simulink model "gap_generation_platoon"  (R2019a)
settings: Solver=VariableStepAuto  StartTime=0.0  StopTime=50  RelTol=1e-3
libraries: simulink x68, powerlib_meascontrol x7, autolibshared x7
(part 2 of 3)

== system gap_generation_platoon/p2 ==
  leaderStates : Inport
  virtualLeaderStates : Inport  Port=2
  lcFlag : Inport  Port=3
  activate ACC-v : Inport  Port=4
  ACC : Subsystem
  ACC-v : Subsystem
  AND : Logic  IconShape=distinctive  AllPortsSameDT=off  OutDataTypeStr=boolean
  Bus Creator : BusCreator  Inputs=4
  Bus Selector : BusSelector  OutputSignals=InertFrm.RearAxl.Disp.X,InertFrm.RearAxl.Disp.Y,InertFrm.RearAxl.Vel.Xdot
  Constant : Constant  Value=0
  Constant1 : Constant  Value=maxAcceleration+1
  Detect steady state : Subsystem
  Gain : Gain  Gain=m/2
  Min : MinMax  Inputs=2
  Mux1 : Mux  Inputs=6
  On Delay : powerlib_meascontrol/Logic/On Delay  DelayType=On delay  delay=1  ic=0  Ts=0
      settings: SourceProductName=Simscape Electrical
  Scope1 : Scope  NumInputPorts=3
  Signal Specification : SignalSpecification  Dimensions=1
  Switch : Switch  Criteria=u2 > Threshold
  Terminator : Terminator
  Triggered Subsystem : Subsystem  TreatAsAtomicUnit=on
  Vehicle Body 3DOF Single Track : autolibshared/Vehicle Body 3DOF Single Track  trackMode=Single (bicycle)  inputMode=External longitudinal forces  frontSteerMode=on  rearSteerMode=off  windMode=off  muMode=off  extFMode=off  extMMode=off  extXo=off  extpsio=off  extxdoto=off  extro=off  extYo=off  extTamb=off  extydoto=off  aMode=2  NF=2  NR=2  m=m  a=lf  b=lr  h=0.35  X_o=x0  xdot_o=vx0  CalphaMode=off  sigmaMode=on  d=0  w=[1.4,1.4]  Cy_f=12e3  Cy_r=11e3  sigma_f=.1  sigma_r=.1  alpha_f_brk=[-.1 .1]  Cy_f_data=[-9e3 9e3]  alpha_r_brk=[-.1 .1]  Cy_r_data=[-9e3 9e3]  Y_o=y0  ydot_o=0  Izz=4000  psi_o=0  r_o=0  Af=2  Cd=.3  Cl=.1  Cpm=.1  beta_w=[0:0.01:0.3]  Cs=[0:0.03:0.9]  Cym=[0:0.01:0.3]  Pabs=101325  Tair=273  g=9.81  mu=1  xdot_tol=.01  Fznom=5000  Fxtire_sat=7e4  Fytire_sat=7e4  longOff=0  latOff=0  vertOff=0  wrapAng=off
      settings: SourceProductName=Powertrain Blockset  SourceProductBaseCode=PW
  states : Outport
  errors : Outport  Port=2
  gap : Outport  Port=3
  virtualErrors : Outport  Port=4
  virtualGap : Outport  Port=5
  gapRequest : Outport  Port=6
  wires:
  Detect steady state/1(Out1) -> AND/1
  Triggered Subsystem/1(Out1) -> gapRequest/1
  On Delay/1 -> AND/2, Triggered Subsystem/1(In1)
  AND/1 -> Triggered Subsystem/Trigger
  Constant1/1 -> Switch/3
  activate ACC-v/1 -> Detect steady state/3(ACC-v active), ACC-v/3(activate), Switch/2
  Signal Specification/1 -> Gain/1, Bus Creator/4
  Bus Selector/2 -> Bus Creator/2  "<Y>"
  ACC-v/3(gap) -> virtualGap/1
  ACC-v/2(errors) -> virtualErrors/1, Detect steady state/2(virtual errors)
  ACC-v/1(u) -> Switch/1
  Switch/1 -> Min/2, Scope1/2  "acc-v"
  lcFlag/1 -> ACC/3(lcFlag), On Delay/1, ACC-v/4(lcFlag)
  ACC/2(errors) -> Detect steady state/1(errors), errors/1
  virtualLeaderStates/1 -> ACC-v/2(leaderStates)
  leaderStates/1 -> ACC/2(leaderStates)
  Bus Creator/1 -> states/1, ACC-v/1(currentStates), ACC/1(currentStates)
  ACC/3(gap) -> gap/1
  Mux1/1 -> Terminator/1
  Vehicle Body 3DOF Single Track/7 -> Mux1/6
  Vehicle Body 3DOF Single Track/6 -> Mux1/5
  Vehicle Body 3DOF Single Track/5 -> Mux1/4
  Vehicle Body 3DOF Single Track/2 -> Mux1/1
  Vehicle Body 3DOF Single Track/3 -> Mux1/2
  Vehicle Body 3DOF Single Track/4 -> Mux1/3
  Vehicle Body 3DOF Single Track/1 -> Bus Selector/1
  Constant/1 -> Vehicle Body 3DOF Single Track/1
  Gain/1 -> Vehicle Body 3DOF Single Track/2, Vehicle Body 3DOF Single Track/3
  ACC/1(u) -> Min/1, Scope1/1  "acc"
  Min/1 -> Signal Specification/1, Scope1/3  "u"
  Bus Selector/1 -> Bus Creator/1  "<X>"
  Bus Selector/3 -> Bus Creator/3  "<Xdot>"

== system gap_generation_platoon/p3 ==
  leaderStates : Inport
  virtualLeaderStates : Inport  Port=2
  lcFlag : Inport  Port=3
  activate ACC-v : Inport  Port=4
  ACC : Subsystem
  ACC-v : Subsystem
  AND : Logic  IconShape=distinctive  AllPortsSameDT=off  OutDataTypeStr=boolean
  Bus Creator : BusCreator  Inputs=4
  Bus Selector : BusSelector  OutputSignals=InertFrm.RearAxl.Disp.X,InertFrm.RearAxl.Disp.Y,InertFrm.RearAxl.Vel.Xdot
  Constant : Constant  Value=0
  Constant1 : Constant  Value=maxAcceleration+1
  Detect steady state : Subsystem
  Gain : Gain  Gain=m/2
  Min : MinMax  Inputs=2
  Mux1 : Mux  Inputs=6
  On Delay : powerlib_meascontrol/Logic/On Delay  DelayType=On delay  delay=1  ic=0  Ts=0
      settings: SourceProductName=Simscape Electrical
  Scope1 : Scope  NumInputPorts=3
  Signal Specification : SignalSpecification  Dimensions=1
  Switch : Switch  Criteria=u2 > Threshold
  Terminator : Terminator
  Triggered Subsystem : Subsystem  TreatAsAtomicUnit=on
  Vehicle Body 3DOF Single Track : autolibshared/Vehicle Body 3DOF Single Track  trackMode=Single (bicycle)  inputMode=External longitudinal forces  frontSteerMode=on  rearSteerMode=off  windMode=off  muMode=off  extFMode=off  extMMode=off  extXo=off  extpsio=off  extxdoto=off  extro=off  extYo=off  extTamb=off  extydoto=off  aMode=2  NF=2  NR=2  m=m  a=lf  b=lr  h=0.35  X_o=x0  xdot_o=vx0  CalphaMode=off  sigmaMode=on  d=0  w=[1.4,1.4]  Cy_f=12e3  Cy_r=11e3  sigma_f=.1  sigma_r=.1  alpha_f_brk=[-.1 .1]  Cy_f_data=[-9e3 9e3]  alpha_r_brk=[-.1 .1]  Cy_r_data=[-9e3 9e3]  Y_o=y0  ydot_o=0  Izz=4000  psi_o=0  r_o=0  Af=2  Cd=.3  Cl=.1  Cpm=.1  beta_w=[0:0.01:0.3]  Cs=[0:0.03:0.9]  Cym=[0:0.01:0.3]  Pabs=101325  Tair=273  g=9.81  mu=1  xdot_tol=.01  Fznom=5000  Fxtire_sat=7e4  Fytire_sat=7e4  longOff=0  latOff=0  vertOff=0  wrapAng=off
      settings: SourceProductName=Powertrain Blockset  SourceProductBaseCode=PW
  states : Outport
  errors : Outport  Port=2
  gap : Outport  Port=3
  virtualErrors : Outport  Port=4
  virtualGap : Outport  Port=5
  gapRequest : Outport  Port=6
  wires:
  Bus Selector/3 -> Bus Creator/3  "<Xdot>"
  Bus Selector/1 -> Bus Creator/1  "<X>"
  Min/1 -> Scope1/3, Signal Specification/1  "u"
  ACC/1(u) -> Scope1/1, Min/1  "acc"
  Gain/1 -> Vehicle Body 3DOF Single Track/3, Vehicle Body 3DOF Single Track/2
  Constant/1 -> Vehicle Body 3DOF Single Track/1
  Vehicle Body 3DOF Single Track/1 -> Bus Selector/1
  Vehicle Body 3DOF Single Track/4 -> Mux1/3
  Vehicle Body 3DOF Single Track/3 -> Mux1/2
  Vehicle Body 3DOF Single Track/2 -> Mux1/1
  Vehicle Body 3DOF Single Track/5 -> Mux1/4
  Vehicle Body 3DOF Single Track/6 -> Mux1/5
  Vehicle Body 3DOF Single Track/7 -> Mux1/6
  Mux1/1 -> Terminator/1
  ACC/3(gap) -> gap/1
  Bus Creator/1 -> ACC/1(currentStates), ACC-v/1(currentStates), states/1
  leaderStates/1 -> ACC/2(leaderStates)
  virtualLeaderStates/1 -> ACC-v/2(leaderStates)
  ACC/2(errors) -> errors/1, Detect steady state/1(errors)
  lcFlag/1 -> ACC-v/4(lcFlag), On Delay/1, ACC/3(lcFlag)
  Switch/1 -> Scope1/2, Min/2  "acc-v"
  ACC-v/1(u) -> Switch/1
  ACC-v/2(errors) -> Detect steady state/2(virtual errors), virtualErrors/1
  ACC-v/3(gap) -> virtualGap/1
  Bus Selector/2 -> Bus Creator/2  "<Y>"
  Signal Specification/1 -> Bus Creator/4, Gain/1
  activate ACC-v/1 -> Switch/2, ACC-v/3(activate), Detect steady state/3(ACC-v active)
  Constant1/1 -> Switch/3
  AND/1 -> Triggered Subsystem/Trigger
  On Delay/1 -> Triggered Subsystem/1(In1), AND/2
  Triggered Subsystem/1(Out1) -> gapRequest/1
  Detect steady state/1(Out1) -> AND/1

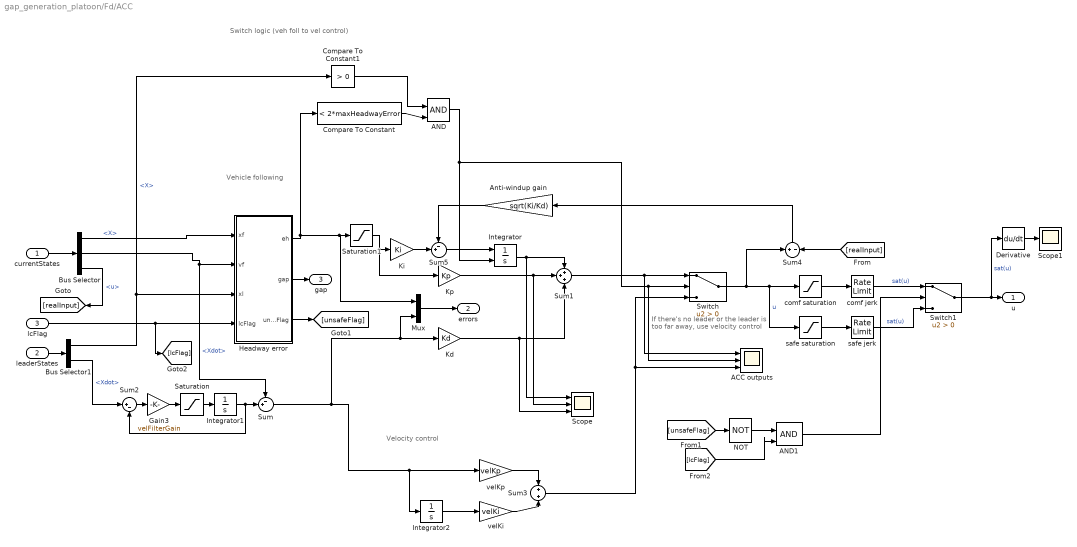
== system gap_generation_platoon/Fd/ACC ==
  note: Vehicle following
  note: Switch logic (veh foll to vel control)
  note: Velocity control
  note: If there's no leader or the leader
      | is too far away, use velocity control
  currentStates : Inport
  leaderStates : Inport  Port=2
  lcFlag : Inport  Port=3
  ACC outputs : Scope  NumInputPorts=3
  AND : Logic  IconShape=distinctive  AllPortsSameDT=off  OutDataTypeStr=boolean
  AND1 : Logic  IconShape=distinctive  AllPortsSameDT=off  OutDataTypeStr=boolean
  Anti-windup gain : Gain  Gain=sqrt(Ki/Kd)
  Bus Selector : BusSelector  OutputSignals=X,Xdot,u
  Bus Selector1 : BusSelector  OutputSignals=X,Xdot
  Compare To Constant : simulink/Logic and Bit Operations/Compare To Constant  relop=<  const=2*maxHeadwayError  OutDataTypeStr=boolean
  Compare To Constant1 : simulink/Logic and Bit Operations/Compare To Constant  relop=>  const=0  OutDataTypeStr=boolean
  Derivative : Derivative
  Gain3 : Gain  Gain=velFilterGain
  Headway error : Subsystem
  Integrator : Integrator  ExternalReset=either
  Integrator1 : Integrator  InitialCondition=vx0
  Integrator2 : Integrator
  Kd : Gain  Gain=Kd
  Ki : Gain  Gain=Ki
  Kp : Gain  Gain=Kp
  Mux : Mux  Inputs=2
  NOT : Logic  Operator=NOT  IconShape=distinctive  AllPortsSameDT=off  OutDataTypeStr=boolean
  Saturation : Saturate  UpperLimit=maxAcceleration  LowerLimit=minAcceleration
  Saturation1 : Saturate  UpperLimit=maxHeadwayError  LowerLimit=minHeadwayError
  Scope : Scope  NumInputPorts=3
  Scope1 : Scope
  Sum : Sum  Inputs=-+|
  Sum1 : Sum  Inputs=+++
  Sum2 : Sum  Inputs=|+-
  Sum3 : Sum
  Sum4 : Sum  Inputs=+-
  Sum5 : Sum  Inputs=-+|
  Switch : Switch  Criteria=u2 > Threshold
  Switch1 : Switch  Criteria=u2 > Threshold
  comf jerk : RateLimiter  RisingSlewLimit=10  FallingSlewLimit=-10  SampleTimeMode=inherited
  comf saturation : Saturate  UpperLimit=maxAcceleration/2  LowerLimit=minAcceleration/4
  safe jerk : RateLimiter  RisingSlewLimit=maxJerk  FallingSlewLimit=minJerk  SampleTimeMode=inherited
  safe saturation : Saturate  UpperLimit=maxAcceleration  LowerLimit=minAcceleration
  velKi : Gain  Gain=velKi
  velKp : Gain  Gain=velKp
  u : Outport
  errors : Outport  Port=2
  gap : Outport  Port=3
  wires:
  Headway error/1(eh) -> Saturation1/1, Mux/1, Compare To Constant/1
  Bus Selector/2 -> Headway error/2(vf), Sum/1  "<Xdot>"
  Kd/1 -> Scope/3, Sum1/3
  Kp/1 -> Scope/2, Sum1/2
  Gain3/1 -> Saturation/1
  Saturation/1 -> Integrator1/1
  Integrator1/1 -> Sum2/2, Sum/2
  Bus Selector1/2 -> Sum2/1  "<Xdot>"
  Sum2/1 -> Gain3/1
  Saturation1/1 -> Kp/1, Ki/1
  Headway error/2("gap ") -> gap/1
  Integrator2/1 -> velKi/1
  velKi/1 -> Sum3/2
  Switch/1 -> Sum4/1, safe saturation/1, comf saturation/1  "u"
  Sum1/1 -> Switch/1, ACC outputs/1
  Sum3/1 -> ACC outputs/3, Switch/3
  Sum/1 -> Mux/2, Kd/1, velKp/1, Integrator2/1
  Mux/1 -> errors/1
  Sum4/1 -> Anti-windup gain/1
  Sum5/1 -> Integrator/1
  Switch1/1 -> Derivative/1, u/1  "sat(u)"
  velKp/1 -> Sum3/1
  Ki/1 -> Sum5/2
  Integrator/1 -> Sum1/1, Scope/1
  Anti-windup gain/1 -> Sum5/1
  AND/1 -> Integrator/2, Switch/2, ACC outputs/2
  Compare To Constant/1 -> AND/2
  Compare To Constant1/1 -> AND/1
  lcFlag/1 -> [lcFlag], Headway error/4(lcFlag)
  currentStates/1 -> Bus Selector/1
  Bus Selector/1 -> Headway error/1(xf)  "<X>"
  leaderStates/1 -> Bus Selector1/1
  Bus Selector1/1 -> Compare To Constant1/1, Headway error/3(xl)  "<X>"
  Bus Selector/3 -> [realInput]  "<u>"
  [realInput] -> Sum4/2
  Headway error/3(unsafeFlag) -> [unsafeFlag]
  [unsafeFlag] -> NOT/1
  NOT/1 -> AND1/1
  [lcFlag] -> AND1/2
  AND1/1 -> Switch1/2
  safe saturation/1 -> safe jerk/1
  comf saturation/1 -> comf jerk/1
  safe jerk/1 -> Switch1/3  "sat(u)"
  comf jerk/1 -> Switch1/1  "sat(u)"
  Derivative/1 -> Scope1/1

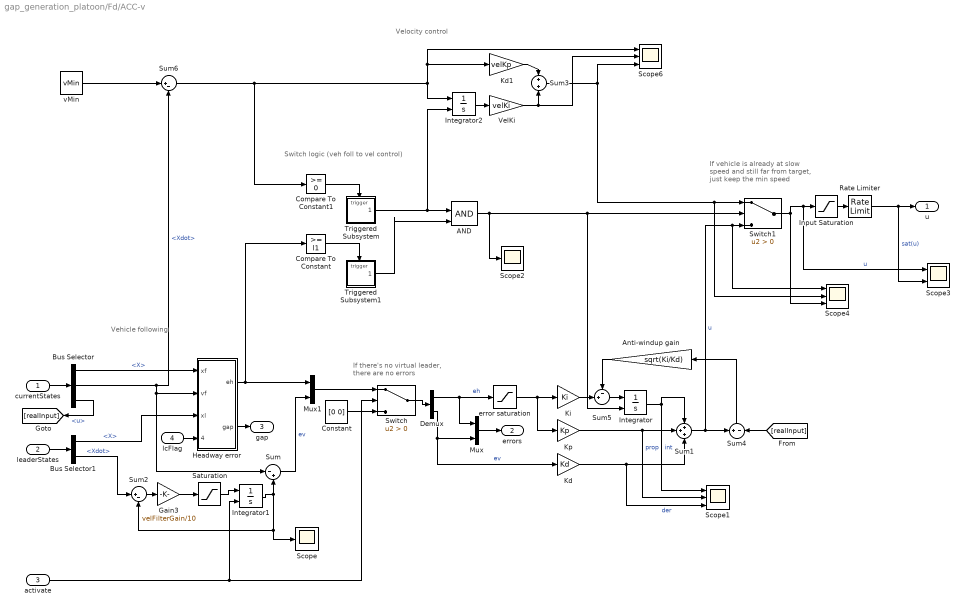
== system gap_generation_platoon/Fd/ACC-v ==
  note: Vehicle following
  note: Switch logic (veh foll to vel control)
  note: Velocity control
  note: If vehicle is already at slow
      | speed and still far from target,
      | just keep the min speed
  note: If there's no virtual leader,
      | there are no errors
  currentStates : Inport
  leaderStates : Inport  Port=2
  activate : Inport  Port=3
  lcFlag : Inport  Port=4
  AND : Logic  IconShape=distinctive  AllPortsSameDT=off  OutDataTypeStr=boolean
  Anti-windup gain : Gain  Gain=sqrt(Ki/Kd)
  Bus Selector : BusSelector  OutputSignals=X,Xdot,u
  Bus Selector1 : BusSelector  OutputSignals=X,Xdot
  Compare To Constant : simulink/Logic and Bit Operations/Compare To Constant  relop=>=  const=l1  OutDataTypeStr=boolean
  Compare To Constant1 : simulink/Logic and Bit Operations/Compare To Constant  relop=>=  const=0  OutDataTypeStr=boolean
  Constant : Constant  Value=[0 0]
  Demux : Demux  Outputs=2
  Gain3 : Gain  Gain=velFilterGain/10
  Headway error : Subsystem
  Input Saturation : Saturate  UpperLimit=maxAcceleration/2  LowerLimit=minAcceleration/4
  Integrator : Integrator  ExternalReset=falling
  Integrator1 : Integrator  ExternalReset=rising  InitialCondition=vx0
  Integrator2 : Integrator  ExternalReset=rising
  Kd : Gain  Gain=Kd
  Kd1 : Gain  Gain=velKp
  Ki : Gain  Gain=Ki
  Kp : Gain  Gain=Kp
  Mux : Mux  Inputs=2
  Mux1 : Mux  Inputs=2
  Rate Limiter : RateLimiter  RisingSlewLimit=10  FallingSlewLimit=-10  SampleTimeMode=inherited
  Saturation : Saturate  UpperLimit=maxAcceleration  LowerLimit=minAcceleration
  Scope : Scope
  Scope1 : Scope  NumInputPorts=3
  Scope2 : Scope
  Scope3 : Scope  NumInputPorts=2
  Scope4 : Scope  NumInputPorts=3
  Scope6 : Scope  NumInputPorts=3
  Sum : Sum  Inputs=|-+
  Sum1 : Sum  Inputs=+++
  Sum2 : Sum  Inputs=|+-
  Sum3 : Sum
  Sum4 : Sum  Inputs=+-
  Sum5 : Sum  Inputs=-+|
  Sum6 : Sum  Inputs=|+-
  Switch : Switch  Criteria=u2 > Threshold
  Switch1 : Switch  Criteria=u2 > Threshold
  Triggered Subsystem : Subsystem  TreatAsAtomicUnit=on
  Triggered Subsystem1 : Subsystem  TreatAsAtomicUnit=on
  VelKi : Gain  Gain=velKi
  error saturation : Saturate  UpperLimit=maxHeadwayError  LowerLimit=minHeadwayError/10
  vMin : Constant  Value=vMin
  u : Outport
  errors : Outport  Port=2
  gap : Outport  Port=3
  wires:
  Headway error/1(eh) -> Mux1/1, Compare To Constant/1
  Kd/1 -> Scope1/3, Sum1/3  "der"
  Kp/1 -> Scope1/2, Sum1/2  "prop"
  Gain3/1 -> Saturation/1
  Saturation/1 -> Integrator1/1
  Integrator1/1 -> Scope/1, Sum2/2, Sum/2
  Bus Selector1/2 -> Sum2/1  "<Xdot>"
  Sum2/1 -> Gain3/1
  Demux/1 -> error saturation/1, Mux/1  "eh"
  Headway error/2("gap ") -> gap/1
  Sum1/1 -> Scope4/1, Switch1/3, Sum4/1  "u"
  Sum/1 -> Mux1/2  "ev"
  Mux/1 -> errors/1
  Input Saturation/1 -> Rate Limiter/1
  Integrator/1 -> Sum1/1, Scope1/1  "int"
  Sum4/1 -> Anti-windup gain/1
  Ki/1 -> Sum5/2
  Anti-windup gain/1 -> Sum5/1
  Demux/2 -> Mux/2, Kd/1  "ev"
  Switch/1 -> Demux/1
  Mux1/1 -> Switch/1
  activate/1 -> Switch/2, Integrator1/2
  Constant/1 -> Switch/3
  Rate Limiter/1 -> Scope3/2, u/1  "sat(u)"
  Compare To Constant1/1 -> Triggered Subsystem/Trigger
  Compare To Constant/1 -> Triggered Subsystem1/Trigger
  Sum6/1 -> Scope6/1, Kd1/1, Integrator2/1, Compare To Constant1/1
  Sum3/1 -> Scope6/3, Scope4/2, Switch1/1
  Integrator2/1 -> VelKi/1
  Kd1/1 -> Sum3/1
  VelKi/1 -> Scope6/2, Sum3/2
  vMin/1 -> Sum6/1
  Switch1/1 -> Scope3/1, Input Saturation/1, Scope4/3  "u"
  error saturation/1 -> Kp/1, Ki/1
  Sum5/1 -> Integrator/1
  Triggered Subsystem/1(Out1) -> AND/1, Integrator2/2
  [realInput] -> Sum4/2
  currentStates/1 -> Bus Selector/1
  Bus Selector/1 -> Headway error/1(xf)  "<X>"
  Bus Selector/2 -> Sum6/2, Headway error/2(vf), Sum/1  "<Xdot>"
  leaderStates/1 -> Bus Selector1/1
  Bus Selector1/1 -> Headway error/3(xl)  "<X>"
  Bus Selector/3 -> [realInput]  "<u>"
  lcFlag/1 -> Headway error/4(lcFlag)
  Triggered Subsystem1/1(Out1) -> AND/2
  AND/1 -> Switch1/2, Integrator/2, Scope2/1

== system gap_generation_platoon/Fd/Triggered Subsystem ==
  In1 : Inport
  Trigger : TriggerPort  VariantControl=Variant
  Out1 : Outport
  wires:
  In1/1 -> Out1/1

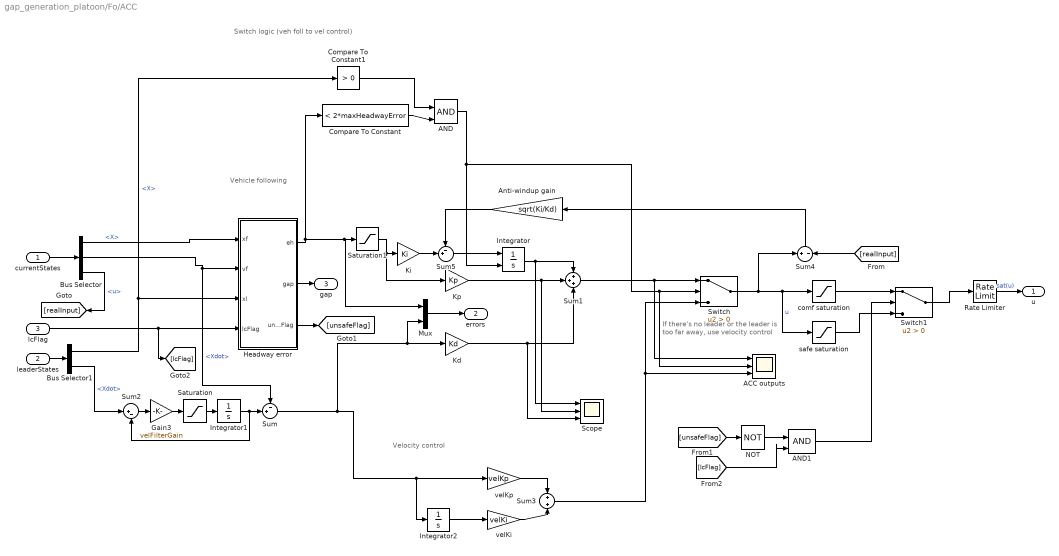
== system gap_generation_platoon/Fo/ACC ==
  note: If there's no leader or the leader
      | is too far away, use velocity control
  note: Velocity control
  note: Switch logic (veh foll to vel control)
  note: Vehicle following
  currentStates : Inport
  leaderStates : Inport  Port=2
  lcFlag : Inport  Port=3
  ACC outputs : Scope  NumInputPorts=3
  AND : Logic  IconShape=distinctive  AllPortsSameDT=off  OutDataTypeStr=boolean
  AND1 : Logic  IconShape=distinctive  AllPortsSameDT=off  OutDataTypeStr=boolean
  Anti-windup gain : Gain  Gain=sqrt(Ki/Kd)
  Bus Selector : BusSelector  OutputSignals=X,Xdot,u
  Bus Selector1 : BusSelector  OutputSignals=X,Xdot
  Compare To Constant : simulink/Logic and Bit Operations/Compare To Constant  relop=<  const=2*maxHeadwayError  OutDataTypeStr=boolean
  Compare To Constant1 : simulink/Logic and Bit Operations/Compare To Constant  relop=>  const=0  OutDataTypeStr=boolean
  Gain3 : Gain  Gain=velFilterGain
  Headway error : Subsystem
  Integrator : Integrator  ExternalReset=either
  Integrator1 : Integrator  InitialCondition=vx0
  Integrator2 : Integrator
  Kd : Gain  Gain=Kd
  Ki : Gain  Gain=Ki
  Kp : Gain  Gain=Kp
  Mux : Mux  Inputs=2
  NOT : Logic  Operator=NOT  IconShape=distinctive  AllPortsSameDT=off  OutDataTypeStr=boolean
  Rate Limiter : RateLimiter  RisingSlewLimit=maxJerk  FallingSlewLimit=minJerk  SampleTimeMode=inherited
  Saturation : Saturate  UpperLimit=maxAcceleration  LowerLimit=minAcceleration
  Saturation1 : Saturate  UpperLimit=maxHeadwayError  LowerLimit=minHeadwayError
  Scope : Scope  NumInputPorts=3
  Sum : Sum  Inputs=-+|
  Sum1 : Sum  Inputs=+++
  Sum2 : Sum  Inputs=|+-
  Sum3 : Sum
  Sum4 : Sum  Inputs=+-
  Sum5 : Sum  Inputs=-+|
  Switch : Switch  Criteria=u2 > Threshold
  Switch1 : Switch  Criteria=u2 > Threshold
  comf saturation : Saturate  UpperLimit=maxAcceleration/2  LowerLimit=minAcceleration/4
  safe saturation : Saturate  UpperLimit=maxAcceleration  LowerLimit=minAcceleration
  velKi : Gain  Gain=velKi
  velKp : Gain  Gain=velKp
  u : Outport
  errors : Outport  Port=2
  gap : Outport  Port=3
  wires:
  comf saturation/1 -> Switch1/1
  safe saturation/1 -> Switch1/3
  Switch1/1 -> Rate Limiter/1
  AND1/1 -> Switch1/2
  [lcFlag] -> AND1/2
  NOT/1 -> AND1/1
  [unsafeFlag] -> NOT/1
  Headway error/3(unsafeFlag) -> [unsafeFlag]
  [realInput] -> Sum4/2
  Bus Selector/3 -> [realInput]  "<u>"
  Bus Selector1/1 -> Headway error/3(xl), Compare To Constant1/1  "<X>"
  leaderStates/1 -> Bus Selector1/1
  Bus Selector/1 -> Headway error/1(xf)  "<X>"
  currentStates/1 -> Bus Selector/1
  lcFlag/1 -> Headway error/4(lcFlag), [lcFlag]
  Compare To Constant1/1 -> AND/1
  Compare To Constant/1 -> AND/2
  AND/1 -> ACC outputs/2, Switch/2, Integrator/2
  Anti-windup gain/1 -> Sum5/1
  Integrator/1 -> Scope/1, Sum1/1
  Ki/1 -> Sum5/2
  velKp/1 -> Sum3/1
  Rate Limiter/1 -> u/1  "sat(u)"
  Sum5/1 -> Integrator/1
  Sum4/1 -> Anti-windup gain/1
  Mux/1 -> errors/1
  Sum/1 -> Integrator2/1, velKp/1, Kd/1, Mux/2
  Sum3/1 -> Switch/3, ACC outputs/3
  Sum1/1 -> ACC outputs/1, Switch/1
  Switch/1 -> comf saturation/1, safe saturation/1, Sum4/1  "u"
  velKi/1 -> Sum3/2
  Integrator2/1 -> velKi/1
  Headway error/2("gap ") -> gap/1
  Saturation1/1 -> Ki/1, Kp/1
  Sum2/1 -> Gain3/1
  Bus Selector1/2 -> Sum2/1  "<Xdot>"
  Integrator1/1 -> Sum/2, Sum2/2
  Saturation/1 -> Integrator1/1
  Gain3/1 -> Saturation/1
  Kp/1 -> Sum1/2, Scope/2
  Kd/1 -> Sum1/3, Scope/3
  Bus Selector/2 -> Sum/1, Headway error/2(vf)  "<Xdot>"
  Headway error/1(eh) -> Compare To Constant/1, Mux/1, Saturation1/1

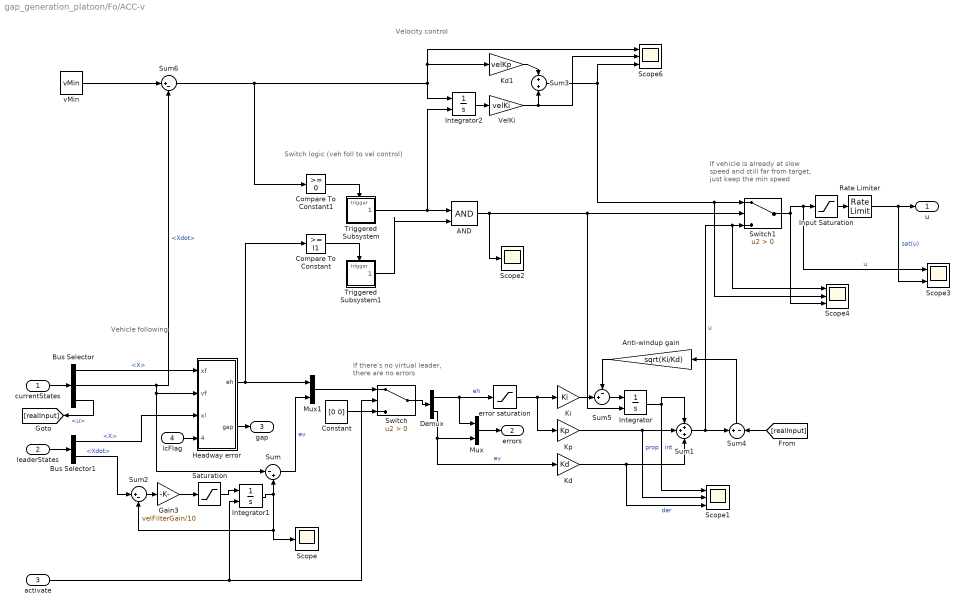
== system gap_generation_platoon/Fo/ACC-v ==
  note: If there's no virtual leader,
      | there are no errors
  note: If vehicle is already at slow
      | speed and still far from target,
      | just keep the min speed
  note: Velocity control
  note: Switch logic (veh foll to vel control)
  note: Vehicle following
  currentStates : Inport
  leaderStates : Inport  Port=2
  activate : Inport  Port=3
  lcFlag : Inport  Port=4
  AND : Logic  IconShape=distinctive  AllPortsSameDT=off  OutDataTypeStr=boolean
  Anti-windup gain : Gain  Gain=sqrt(Ki/Kd)
  Bus Selector : BusSelector  OutputSignals=X,Xdot,u
  Bus Selector1 : BusSelector  OutputSignals=X,Xdot
  Compare To Constant : simulink/Logic and Bit Operations/Compare To Constant  relop=>=  const=l1  OutDataTypeStr=boolean
  Compare To Constant1 : simulink/Logic and Bit Operations/Compare To Constant  relop=>=  const=0  OutDataTypeStr=boolean
  Constant : Constant  Value=[0 0]
  Demux : Demux  Outputs=2
  Gain3 : Gain  Gain=velFilterGain/10
  Headway error : Subsystem
  Input Saturation : Saturate  UpperLimit=maxAcceleration/2  LowerLimit=minAcceleration/4
  Integrator : Integrator  ExternalReset=falling
  Integrator1 : Integrator  ExternalReset=rising  InitialCondition=vx0
  Integrator2 : Integrator  ExternalReset=rising
  Kd : Gain  Gain=Kd
  Kd1 : Gain  Gain=velKp
  Ki : Gain  Gain=Ki
  Kp : Gain  Gain=Kp
  Mux : Mux  Inputs=2
  Mux1 : Mux  Inputs=2
  Rate Limiter : RateLimiter  RisingSlewLimit=maxJerk/2  FallingSlewLimit=minJerk/3  SampleTimeMode=inherited
  Saturation : Saturate  UpperLimit=maxAcceleration  LowerLimit=minAcceleration
  Scope : Scope
  Scope1 : Scope  NumInputPorts=3
  Scope2 : Scope
  Scope3 : Scope  NumInputPorts=2
  Scope4 : Scope  NumInputPorts=3
  Scope6 : Scope  NumInputPorts=3
  Sum : Sum  Inputs=|-+
  Sum1 : Sum  Inputs=+++
  Sum2 : Sum  Inputs=|+-
  Sum3 : Sum
  Sum4 : Sum  Inputs=+-
  Sum5 : Sum  Inputs=-+|
  Sum6 : Sum  Inputs=|+-
  Switch : Switch  Criteria=u2 > Threshold
  Switch1 : Switch  Criteria=u2 > Threshold
  Triggered Subsystem : Subsystem  TreatAsAtomicUnit=on
  Triggered Subsystem1 : Subsystem  TreatAsAtomicUnit=on
  VelKi : Gain  Gain=velKi
  error saturation : Saturate  UpperLimit=maxHeadwayError  LowerLimit=minHeadwayError/10
  vMin : Constant  Value=vMin
  u : Outport
  errors : Outport  Port=2
  gap : Outport  Port=3
  wires:
  AND/1 -> Scope2/1, Integrator/2, Switch1/2
  Triggered Subsystem1/1(Out1) -> AND/2
  lcFlag/1 -> Headway error/4(lcFlag)
  Bus Selector/3 -> [realInput]  "<u>"
  Bus Selector1/1 -> Headway error/3(xl)  "<X>"
  leaderStates/1 -> Bus Selector1/1
  Bus Selector/2 -> Sum/1, Headway error/2(vf), Sum6/2  "<Xdot>"
  Bus Selector/1 -> Headway error/1(xf)  "<X>"
  currentStates/1 -> Bus Selector/1
  [realInput] -> Sum4/2
  Triggered Subsystem/1(Out1) -> Integrator2/2, AND/1
  Sum5/1 -> Integrator/1
  error saturation/1 -> Ki/1, Kp/1
  Switch1/1 -> Scope4/3, Input Saturation/1, Scope3/1  "u"
  vMin/1 -> Sum6/1
  VelKi/1 -> Sum3/2, Scope6/2
  Kd1/1 -> Sum3/1
  Integrator2/1 -> VelKi/1
  Sum3/1 -> Switch1/1, Scope4/2, Scope6/3
  Sum6/1 -> Compare To Constant1/1, Integrator2/1, Kd1/1, Scope6/1
  Compare To Constant/1 -> Triggered Subsystem1/Trigger
  Compare To Constant1/1 -> Triggered Subsystem/Trigger
  Rate Limiter/1 -> u/1, Scope3/2  "sat(u)"
  Constant/1 -> Switch/3
  activate/1 -> Integrator1/2, Switch/2
  Mux1/1 -> Switch/1
  Switch/1 -> Demux/1
  Demux/2 -> Kd/1, Mux/2  "ev"
  Anti-windup gain/1 -> Sum5/1
  Ki/1 -> Sum5/2
  Sum4/1 -> Anti-windup gain/1
  Integrator/1 -> Scope1/1, Sum1/1  "int"
  Input Saturation/1 -> Rate Limiter/1
  Mux/1 -> errors/1
  Sum/1 -> Mux1/2  "ev"
  Sum1/1 -> Sum4/1, Switch1/3, Scope4/1  "u"
  Headway error/2("gap ") -> gap/1
  Demux/1 -> Mux/1, error saturation/1  "eh"
  Sum2/1 -> Gain3/1
  Bus Selector1/2 -> Sum2/1  "<Xdot>"
  Integrator1/1 -> Sum/2, Sum2/2, Scope/1
  Saturation/1 -> Integrator1/1
  Gain3/1 -> Saturation/1
  Kp/1 -> Sum1/2, Scope1/2  "prop"
  Kd/1 -> Sum1/3, Scope1/3  "der"
  Headway error/1(eh) -> Compare To Constant/1, Mux1/1

== system gap_generation_platoon/Fo/Triggered Subsystem ==
  In1 : Inport
  Trigger : TriggerPort  VariantControl=Variant
  Out1 : Outport
  wires:
  In1/1 -> Out1/1

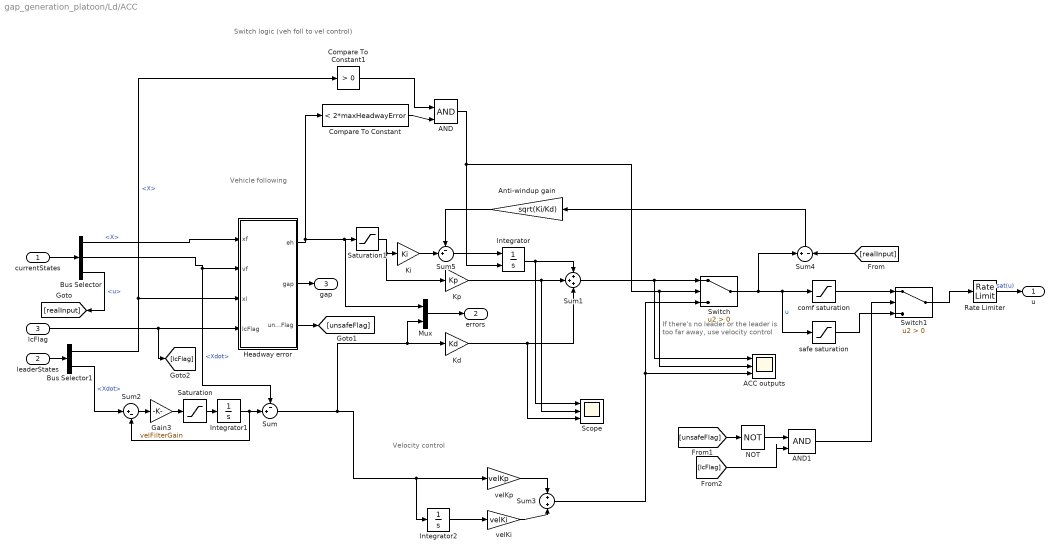
== system gap_generation_platoon/Ld/ACC ==
  note: If there's no leader or the leader
      | is too far away, use velocity control
  note: Velocity control
  note: Switch logic (veh foll to vel control)
  note: Vehicle following
  currentStates : Inport
  leaderStates : Inport  Port=2
  lcFlag : Inport  Port=3
  ACC outputs : Scope  NumInputPorts=3
  AND : Logic  IconShape=distinctive  AllPortsSameDT=off  OutDataTypeStr=boolean
  AND1 : Logic  IconShape=distinctive  AllPortsSameDT=off  OutDataTypeStr=boolean
  Anti-windup gain : Gain  Gain=sqrt(Ki/Kd)
  Bus Selector : BusSelector  OutputSignals=X,Xdot,u
  Bus Selector1 : BusSelector  OutputSignals=X,Xdot
  Compare To Constant : simulink/Logic and Bit Operations/Compare To Constant  relop=<  const=2*maxHeadwayError  OutDataTypeStr=boolean
  Compare To Constant1 : simulink/Logic and Bit Operations/Compare To Constant  relop=>  const=0  OutDataTypeStr=boolean
  Gain3 : Gain  Gain=velFilterGain
  Headway error : Subsystem
  Integrator : Integrator  ExternalReset=either
  Integrator1 : Integrator  InitialCondition=vx0
  Integrator2 : Integrator
  Kd : Gain  Gain=Kd
  Ki : Gain  Gain=Ki
  Kp : Gain  Gain=Kp
  Mux : Mux  Inputs=2
  NOT : Logic  Operator=NOT  IconShape=distinctive  AllPortsSameDT=off  OutDataTypeStr=boolean
  Rate Limiter : RateLimiter  RisingSlewLimit=maxJerk  FallingSlewLimit=minJerk  SampleTimeMode=inherited
  Saturation : Saturate  UpperLimit=maxAcceleration  LowerLimit=minAcceleration
  Saturation1 : Saturate  UpperLimit=maxHeadwayError  LowerLimit=minHeadwayError
  Scope : Scope  NumInputPorts=3
  Sum : Sum  Inputs=-+|
  Sum1 : Sum  Inputs=+++
  Sum2 : Sum  Inputs=|+-
  Sum3 : Sum
  Sum4 : Sum  Inputs=+-
  Sum5 : Sum  Inputs=-+|
  Switch : Switch  Criteria=u2 > Threshold
  Switch1 : Switch  Criteria=u2 > Threshold
  comf saturation : Saturate  UpperLimit=maxAcceleration/2  LowerLimit=minAcceleration/4
  safe saturation : Saturate  UpperLimit=maxAcceleration  LowerLimit=minAcceleration
  velKi : Gain  Gain=velKi
  velKp : Gain  Gain=velKp
  u : Outport
  errors : Outport  Port=2
  gap : Outport  Port=3
  wires:
  comf saturation/1 -> Switch1/1
  safe saturation/1 -> Switch1/3
  Switch1/1 -> Rate Limiter/1
  AND1/1 -> Switch1/2
  [lcFlag] -> AND1/2
  NOT/1 -> AND1/1
  [unsafeFlag] -> NOT/1
  Headway error/3(unsafeFlag) -> [unsafeFlag]
  [realInput] -> Sum4/2
  Bus Selector/3 -> [realInput]  "<u>"
  Bus Selector1/1 -> Headway error/3(xl), Compare To Constant1/1  "<X>"
  leaderStates/1 -> Bus Selector1/1
  Bus Selector/1 -> Headway error/1(xf)  "<X>"
  currentStates/1 -> Bus Selector/1
  lcFlag/1 -> Headway error/4(lcFlag), [lcFlag]
  Compare To Constant1/1 -> AND/1
  Compare To Constant/1 -> AND/2
  AND/1 -> ACC outputs/2, Switch/2, Integrator/2
  Anti-windup gain/1 -> Sum5/1
  Integrator/1 -> Scope/1, Sum1/1
  Ki/1 -> Sum5/2
  velKp/1 -> Sum3/1
  Rate Limiter/1 -> u/1  "sat(u)"
  Sum5/1 -> Integrator/1
  Sum4/1 -> Anti-windup gain/1
  Mux/1 -> errors/1
  Sum/1 -> Integrator2/1, velKp/1, Kd/1, Mux/2
  Sum3/1 -> Switch/3, ACC outputs/3
  Sum1/1 -> ACC outputs/1, Switch/1
  Switch/1 -> comf saturation/1, safe saturation/1, Sum4/1  "u"
  velKi/1 -> Sum3/2
  Integrator2/1 -> velKi/1
  Headway error/2("gap ") -> gap/1
  Saturation1/1 -> Ki/1, Kp/1
  Sum2/1 -> Gain3/1
  Bus Selector1/2 -> Sum2/1  "<Xdot>"
  Integrator1/1 -> Sum/2, Sum2/2
  Saturation/1 -> Integrator1/1
  Gain3/1 -> Saturation/1
  Kp/1 -> Sum1/2, Scope/2
  Kd/1 -> Sum1/3, Scope/3
  Bus Selector/2 -> Sum/1, Headway error/2(vf)  "<Xdot>"
  Headway error/1(eh) -> Compare To Constant/1, Mux/1, Saturation1/1

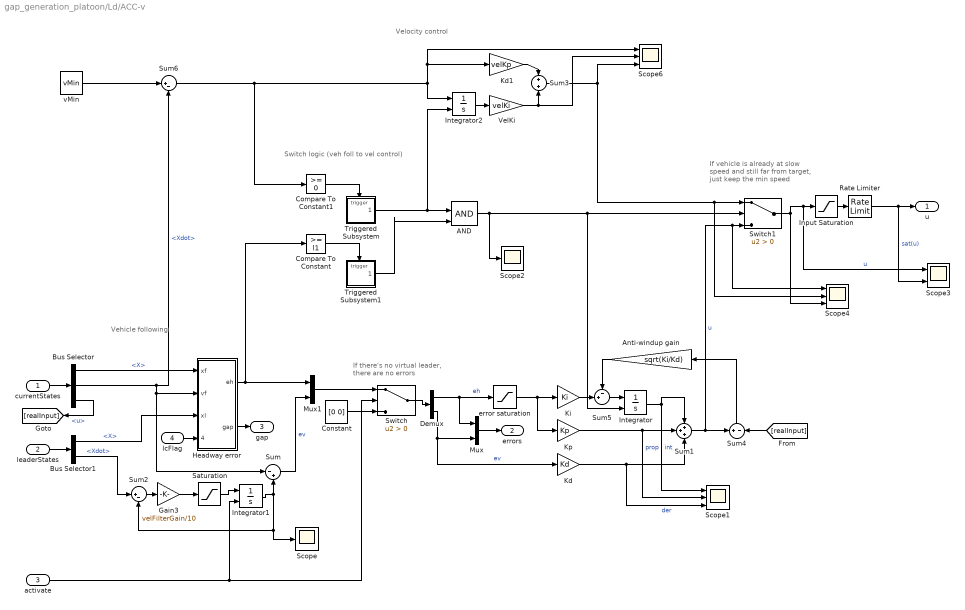
== system gap_generation_platoon/Ld/ACC-v ==
  note: If there's no virtual leader,
      | there are no errors
  note: If vehicle is already at slow
      | speed and still far from target,
      | just keep the min speed
  note: Velocity control
  note: Switch logic (veh foll to vel control)
  note: Vehicle following
  currentStates : Inport
  leaderStates : Inport  Port=2
  activate : Inport  Port=3
  lcFlag : Inport  Port=4
  AND : Logic  IconShape=distinctive  AllPortsSameDT=off  OutDataTypeStr=boolean
  Anti-windup gain : Gain  Gain=sqrt(Ki/Kd)
  Bus Selector : BusSelector  OutputSignals=X,Xdot,u
  Bus Selector1 : BusSelector  OutputSignals=X,Xdot
  Compare To Constant : simulink/Logic and Bit Operations/Compare To Constant  relop=>=  const=l1  OutDataTypeStr=boolean
  Compare To Constant1 : simulink/Logic and Bit Operations/Compare To Constant  relop=>=  const=0  OutDataTypeStr=boolean
  Constant : Constant  Value=[0 0]
  Demux : Demux  Outputs=2
  Gain3 : Gain  Gain=velFilterGain/10
  Headway error : Subsystem
  Input Saturation : Saturate  UpperLimit=maxAcceleration/2  LowerLimit=minAcceleration/4
  Integrator : Integrator  ExternalReset=falling
  Integrator1 : Integrator  ExternalReset=rising  InitialCondition=vx0
  Integrator2 : Integrator  ExternalReset=rising
  Kd : Gain  Gain=Kd
  Kd1 : Gain  Gain=velKp
  Ki : Gain  Gain=Ki
  Kp : Gain  Gain=Kp
  Mux : Mux  Inputs=2
  Mux1 : Mux  Inputs=2
  Rate Limiter : RateLimiter  RisingSlewLimit=maxJerk/2  FallingSlewLimit=minJerk/3  SampleTimeMode=inherited
  Saturation : Saturate  UpperLimit=maxAcceleration  LowerLimit=minAcceleration
  Scope : Scope
  Scope1 : Scope  NumInputPorts=3
  Scope2 : Scope
  Scope3 : Scope  NumInputPorts=2
  Scope4 : Scope  NumInputPorts=3
  Scope6 : Scope  NumInputPorts=3
  Sum : Sum  Inputs=|-+
  Sum1 : Sum  Inputs=+++
  Sum2 : Sum  Inputs=|+-
  Sum3 : Sum
  Sum4 : Sum  Inputs=+-
  Sum5 : Sum  Inputs=-+|
  Sum6 : Sum  Inputs=|+-
  Switch : Switch  Criteria=u2 > Threshold
  Switch1 : Switch  Criteria=u2 > Threshold
  Triggered Subsystem : Subsystem  TreatAsAtomicUnit=on
  Triggered Subsystem1 : Subsystem  TreatAsAtomicUnit=on
  VelKi : Gain  Gain=velKi
  error saturation : Saturate  UpperLimit=maxHeadwayError  LowerLimit=minHeadwayError/10
  vMin : Constant  Value=vMin
  u : Outport
  errors : Outport  Port=2
  gap : Outport  Port=3
  wires:
  AND/1 -> Scope2/1, Integrator/2, Switch1/2
  Triggered Subsystem1/1(Out1) -> AND/2
  lcFlag/1 -> Headway error/4(lcFlag)
  Bus Selector/3 -> [realInput]  "<u>"
  Bus Selector1/1 -> Headway error/3(xl)  "<X>"
  leaderStates/1 -> Bus Selector1/1
  Bus Selector/2 -> Sum/1, Headway error/2(vf), Sum6/2  "<Xdot>"
  Bus Selector/1 -> Headway error/1(xf)  "<X>"
  currentStates/1 -> Bus Selector/1
  [realInput] -> Sum4/2
  Triggered Subsystem/1(Out1) -> Integrator2/2, AND/1
  Sum5/1 -> Integrator/1
  error saturation/1 -> Ki/1, Kp/1
  Switch1/1 -> Scope4/3, Input Saturation/1, Scope3/1  "u"
  vMin/1 -> Sum6/1
  VelKi/1 -> Sum3/2, Scope6/2
  Kd1/1 -> Sum3/1
  Integrator2/1 -> VelKi/1
  Sum3/1 -> Switch1/1, Scope4/2, Scope6/3
  Sum6/1 -> Compare To Constant1/1, Integrator2/1, Kd1/1, Scope6/1
  Compare To Constant/1 -> Triggered Subsystem1/Trigger
  Compare To Constant1/1 -> Triggered Subsystem/Trigger
  Rate Limiter/1 -> u/1, Scope3/2  "sat(u)"
  Constant/1 -> Switch/3
  activate/1 -> Integrator1/2, Switch/2
  Mux1/1 -> Switch/1
  Switch/1 -> Demux/1
  Demux/2 -> Kd/1, Mux/2  "ev"
  Anti-windup gain/1 -> Sum5/1
  Ki/1 -> Sum5/2
  Sum4/1 -> Anti-windup gain/1
  Integrator/1 -> Scope1/1, Sum1/1  "int"
  Input Saturation/1 -> Rate Limiter/1
  Mux/1 -> errors/1
  Sum/1 -> Mux1/2  "ev"
  Sum1/1 -> Sum4/1, Switch1/3, Scope4/1  "u"
  Headway error/2("gap ") -> gap/1
  Demux/1 -> Mux/1, error saturation/1  "eh"
  Sum2/1 -> Gain3/1
  Bus Selector1/2 -> Sum2/1  "<Xdot>"
  Integrator1/1 -> Sum/2, Sum2/2, Scope/1
  Saturation/1 -> Integrator1/1
  Gain3/1 -> Saturation/1
  Kp/1 -> Sum1/2, Scope1/2  "prop"
  Kd/1 -> Sum1/3, Scope1/3  "der"
  Headway error/1(eh) -> Compare To Constant/1, Mux1/1

== system gap_generation_platoon/Ld/Triggered Subsystem ==
  In1 : Inport
  Trigger : TriggerPort  VariantControl=Variant
  Out1 : Outport
  wires:
  In1/1 -> Out1/1

== system gap_generation_platoon/Lo/ACC ==
  note: Vehicle following
  note: Switch logic (veh foll to vel control)
  note: Velocity control
  note: If there's no leader or the leader
      | is too far away, use velocity control
  currentStates : Inport
  leaderStates : Inport  Port=2
  lcFlag : Inport  Port=3
  ACC outputs : Scope  NumInputPorts=3
  AND : Logic  IconShape=distinctive  AllPortsSameDT=off  OutDataTypeStr=boolean
  AND1 : Logic  IconShape=distinctive  AllPortsSameDT=off  OutDataTypeStr=boolean
  Anti-windup gain : Gain  Gain=sqrt(Ki/Kd)
  Bus Selector : BusSelector  OutputSignals=X,Xdot,u
  Bus Selector1 : BusSelector  OutputSignals=X,Xdot
  Compare To Constant : simulink/Logic and Bit Operations/Compare To Constant  relop=<  const=2*maxHeadwayError  OutDataTypeStr=boolean
  Compare To Constant1 : simulink/Logic and Bit Operations/Compare To Constant  relop=>  const=0  OutDataTypeStr=boolean
  Gain3 : Gain  Gain=velFilterGain
  Headway error : Subsystem
  Integrator : Integrator  ExternalReset=either
  Integrator1 : Integrator  InitialCondition=vx0
  Integrator2 : Integrator
  Kd : Gain  Gain=Kd
  Ki : Gain  Gain=Ki
  Kp : Gain  Gain=Kp
  Mux : Mux  Inputs=2
  NOT : Logic  Operator=NOT  IconShape=distinctive  AllPortsSameDT=off  OutDataTypeStr=boolean
  Rate Limiter : RateLimiter  RisingSlewLimit=maxJerk  FallingSlewLimit=minJerk  SampleTimeMode=inherited
  Saturation : Saturate  UpperLimit=maxAcceleration  LowerLimit=minAcceleration
  Saturation1 : Saturate  UpperLimit=maxHeadwayError  LowerLimit=minHeadwayError
  Scope : Scope  NumInputPorts=3
  Sum : Sum  Inputs=-+|
  Sum1 : Sum  Inputs=+++
  Sum2 : Sum  Inputs=|+-
  Sum3 : Sum
  Sum4 : Sum  Inputs=+-
  Sum5 : Sum  Inputs=-+|
  Switch : Switch  Criteria=u2 > Threshold
  Switch1 : Switch  Criteria=u2 > Threshold
  comf saturation : Saturate  UpperLimit=maxAcceleration/2  LowerLimit=minAcceleration/4
  safe saturation : Saturate  UpperLimit=maxAcceleration  LowerLimit=minAcceleration
  velKi : Gain  Gain=velKi
  velKp : Gain  Gain=velKp
  u : Outport
  errors : Outport  Port=2
  gap : Outport  Port=3
  wires:
  Headway error/1(eh) -> Saturation1/1, Mux/1, Compare To Constant/1
  Bus Selector/2 -> Headway error/2(vf), Sum/1  "<Xdot>"
  Kd/1 -> Scope/3, Sum1/3
  Kp/1 -> Scope/2, Sum1/2
  Gain3/1 -> Saturation/1
  Saturation/1 -> Integrator1/1
  Integrator1/1 -> Sum2/2, Sum/2
  Bus Selector1/2 -> Sum2/1  "<Xdot>"
  Sum2/1 -> Gain3/1
  Saturation1/1 -> Kp/1, Ki/1
  Headway error/2("gap ") -> gap/1
  Integrator2/1 -> velKi/1
  velKi/1 -> Sum3/2
  Switch/1 -> Sum4/1, safe saturation/1, comf saturation/1  "u"
  Sum1/1 -> Switch/1, ACC outputs/1
  Sum3/1 -> ACC outputs/3, Switch/3
  Sum/1 -> Mux/2, Kd/1, velKp/1, Integrator2/1
  Mux/1 -> errors/1
  Sum4/1 -> Anti-windup gain/1
  Sum5/1 -> Integrator/1
  Rate Limiter/1 -> u/1  "sat(u)"
  velKp/1 -> Sum3/1
  Ki/1 -> Sum5/2
  Integrator/1 -> Sum1/1, Scope/1
  Anti-windup gain/1 -> Sum5/1
  AND/1 -> Integrator/2, Switch/2, ACC outputs/2
  Compare To Constant/1 -> AND/2
  Compare To Constant1/1 -> AND/1
  lcFlag/1 -> [lcFlag], Headway error/4(lcFlag)
  currentStates/1 -> Bus Selector/1
  Bus Selector/1 -> Headway error/1(xf)  "<X>"
  leaderStates/1 -> Bus Selector1/1
  Bus Selector1/1 -> Compare To Constant1/1, Headway error/3(xl)  "<X>"
  Bus Selector/3 -> [realInput]  "<u>"
  [realInput] -> Sum4/2
  Headway error/3(unsafeFlag) -> [unsafeFlag]
  [unsafeFlag] -> NOT/1
  NOT/1 -> AND1/1
  [lcFlag] -> AND1/2
  AND1/1 -> Switch1/2
  Switch1/1 -> Rate Limiter/1
  safe saturation/1 -> Switch1/3
  comf saturation/1 -> Switch1/1

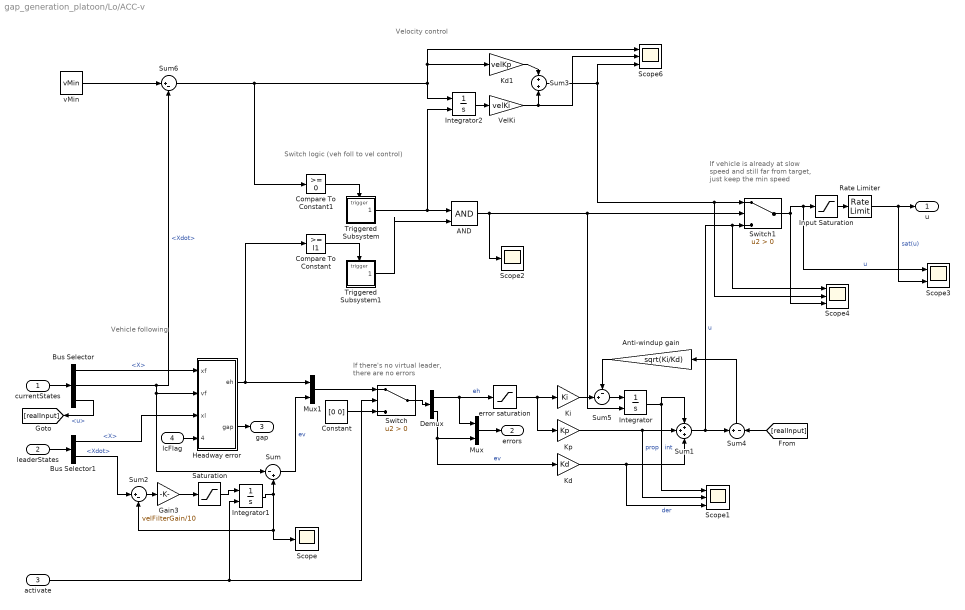
== system gap_generation_platoon/Lo/ACC-v ==
  note: Vehicle following
  note: Switch logic (veh foll to vel control)
  note: Velocity control
  note: If vehicle is already at slow
      | speed and still far from target,
      | just keep the min speed
  note: If there's no virtual leader,
      | there are no errors
  currentStates : Inport
  leaderStates : Inport  Port=2
  activate : Inport  Port=3
  lcFlag : Inport  Port=4
  AND : Logic  IconShape=distinctive  AllPortsSameDT=off  OutDataTypeStr=boolean
  Anti-windup gain : Gain  Gain=sqrt(Ki/Kd)
  Bus Selector : BusSelector  OutputSignals=X,Xdot,u
  Bus Selector1 : BusSelector  OutputSignals=X,Xdot
  Compare To Constant : simulink/Logic and Bit Operations/Compare To Constant  relop=>=  const=l1  OutDataTypeStr=boolean
  Compare To Constant1 : simulink/Logic and Bit Operations/Compare To Constant  relop=>=  const=0  OutDataTypeStr=boolean
  Constant : Constant  Value=[0 0]
  Demux : Demux  Outputs=2
  Gain3 : Gain  Gain=velFilterGain/10
  Headway error : Subsystem
  Input Saturation : Saturate  UpperLimit=maxAcceleration/2  LowerLimit=minAcceleration/4
  Integrator : Integrator  ExternalReset=falling
  Integrator1 : Integrator  ExternalReset=rising  InitialCondition=vx0
  Integrator2 : Integrator  ExternalReset=rising
  Kd : Gain  Gain=Kd
  Kd1 : Gain  Gain=velKp
  Ki : Gain  Gain=Ki
  Kp : Gain  Gain=Kp
  Mux : Mux  Inputs=2
  Mux1 : Mux  Inputs=2
  Rate Limiter : RateLimiter  RisingSlewLimit=maxJerk/2  FallingSlewLimit=minJerk/3  SampleTimeMode=inherited
  Saturation : Saturate  UpperLimit=maxAcceleration  LowerLimit=minAcceleration
  Scope : Scope
  Scope1 : Scope  NumInputPorts=3
  Scope2 : Scope
  Scope3 : Scope  NumInputPorts=2
  Scope4 : Scope  NumInputPorts=3
  Scope6 : Scope  NumInputPorts=3
  Sum : Sum  Inputs=|-+
  Sum1 : Sum  Inputs=+++
  Sum2 : Sum  Inputs=|+-
  Sum3 : Sum
  Sum4 : Sum  Inputs=+-
  Sum5 : Sum  Inputs=-+|
  Sum6 : Sum  Inputs=|+-
  Switch : Switch  Criteria=u2 > Threshold
  Switch1 : Switch  Criteria=u2 > Threshold
  Triggered Subsystem : Subsystem  TreatAsAtomicUnit=on
  Triggered Subsystem1 : Subsystem  TreatAsAtomicUnit=on
  VelKi : Gain  Gain=velKi
  error saturation : Saturate  UpperLimit=maxHeadwayError  LowerLimit=minHeadwayError/10
  vMin : Constant  Value=vMin
  u : Outport
  errors : Outport  Port=2
  gap : Outport  Port=3
  wires:
  Headway error/1(eh) -> Mux1/1, Compare To Constant/1
  Kd/1 -> Scope1/3, Sum1/3  "der"
  Kp/1 -> Scope1/2, Sum1/2  "prop"
  Gain3/1 -> Saturation/1
  Saturation/1 -> Integrator1/1
  Integrator1/1 -> Scope/1, Sum2/2, Sum/2
  Bus Selector1/2 -> Sum2/1  "<Xdot>"
  Sum2/1 -> Gain3/1
  Demux/1 -> error saturation/1, Mux/1  "eh"
  Headway error/2("gap ") -> gap/1
  Sum1/1 -> Scope4/1, Switch1/3, Sum4/1  "u"
  Sum/1 -> Mux1/2  "ev"
  Mux/1 -> errors/1
  Input Saturation/1 -> Rate Limiter/1
  Integrator/1 -> Sum1/1, Scope1/1  "int"
  Sum4/1 -> Anti-windup gain/1
  Ki/1 -> Sum5/2
  Anti-windup gain/1 -> Sum5/1
  Demux/2 -> Mux/2, Kd/1  "ev"
  Switch/1 -> Demux/1
  Mux1/1 -> Switch/1
  activate/1 -> Switch/2, Integrator1/2
  Constant/1 -> Switch/3
  Rate Limiter/1 -> Scope3/2, u/1  "sat(u)"
  Compare To Constant1/1 -> Triggered Subsystem/Trigger
  Compare To Constant/1 -> Triggered Subsystem1/Trigger
  Sum6/1 -> Scope6/1, Kd1/1, Integrator2/1, Compare To Constant1/1
  Sum3/1 -> Scope6/3, Scope4/2, Switch1/1
  Integrator2/1 -> VelKi/1
  Kd1/1 -> Sum3/1
  VelKi/1 -> Scope6/2, Sum3/2
  vMin/1 -> Sum6/1
  Switch1/1 -> Scope3/1, Input Saturation/1, Scope4/3  "u"
  error saturation/1 -> Kp/1, Ki/1
  Sum5/1 -> Integrator/1
  Triggered Subsystem/1(Out1) -> AND/1, Integrator2/2
  [realInput] -> Sum4/2
  currentStates/1 -> Bus Selector/1
  Bus Selector/1 -> Headway error/1(xf)  "<X>"
  Bus Selector/2 -> Sum6/2, Headway error/2(vf), Sum/1  "<Xdot>"
  leaderStates/1 -> Bus Selector1/1
  Bus Selector1/1 -> Headway error/3(xl)  "<X>"
  Bus Selector/3 -> [realInput]  "<u>"
  lcFlag/1 -> Headway error/4(lcFlag)
  Triggered Subsystem1/1(Out1) -> AND/2
  AND/1 -> Switch1/2, Integrator/2, Scope2/1

== system gap_generation_platoon/Lo/Triggered Subsystem ==
  In1 : Inport
  Trigger : TriggerPort  VariantControl=Variant
  Out1 : Outport
  wires:
  In1/1 -> Out1/1

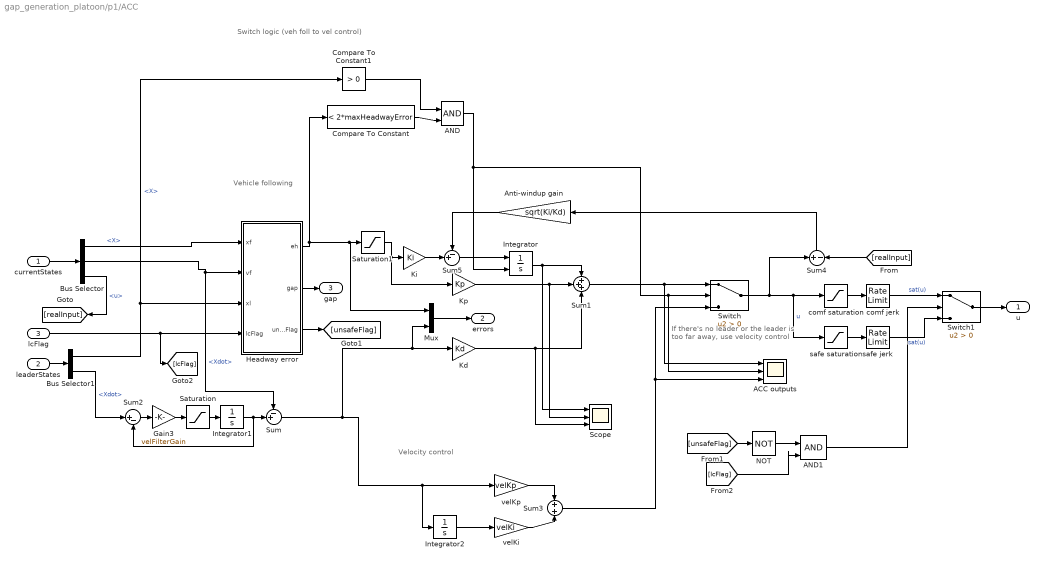
== system gap_generation_platoon/p1/ACC ==
  note: Vehicle following
  note: Switch logic (veh foll to vel control)
  note: Velocity control
  note: If there's no leader or the leader
      | is too far away, use velocity control
  currentStates : Inport
  leaderStates : Inport  Port=2
  lcFlag : Inport  Port=3
  ACC outputs : Scope  NumInputPorts=3
  AND : Logic  IconShape=distinctive  AllPortsSameDT=off  OutDataTypeStr=boolean
  AND1 : Logic  IconShape=distinctive  AllPortsSameDT=off  OutDataTypeStr=boolean
  Anti-windup gain : Gain  Gain=sqrt(Ki/Kd)
  Bus Selector : BusSelector  OutputSignals=X,Xdot,u
  Bus Selector1 : BusSelector  OutputSignals=X,Xdot
  Compare To Constant : simulink/Logic and Bit Operations/Compare To Constant  relop=<  const=2*maxHeadwayError  OutDataTypeStr=boolean
  Compare To Constant1 : simulink/Logic and Bit Operations/Compare To Constant  relop=>  const=0  OutDataTypeStr=boolean
  Gain3 : Gain  Gain=velFilterGain
  Headway error : Subsystem
  Integrator : Integrator  ExternalReset=either
  Integrator1 : Integrator  InitialCondition=vx0
  Integrator2 : Integrator
  Kd : Gain  Gain=Kd
  Ki : Gain  Gain=Ki
  Kp : Gain  Gain=Kp
  Mux : Mux  Inputs=2
  NOT : Logic  Operator=NOT  IconShape=distinctive  AllPortsSameDT=off  OutDataTypeStr=boolean
  Saturation : Saturate  UpperLimit=maxAcceleration  LowerLimit=minAcceleration
  Saturation1 : Saturate  UpperLimit=maxHeadwayError  LowerLimit=minHeadwayError
  Scope : Scope  NumInputPorts=3
  Sum : Sum  Inputs=-+|
  Sum1 : Sum  Inputs=+++
  Sum2 : Sum  Inputs=|+-
  Sum3 : Sum
  Sum4 : Sum  Inputs=+-
  Sum5 : Sum  Inputs=-+|
  Switch : Switch  Criteria=u2 > Threshold
  Switch1 : Switch  Criteria=u2 > Threshold
  comf jerk : RateLimiter  RisingSlewLimit=10  FallingSlewLimit=-10  SampleTimeMode=inherited
  comf saturation : Saturate  UpperLimit=maxAcceleration/2  LowerLimit=minAcceleration/4
  safe jerk : RateLimiter  RisingSlewLimit=maxJerk  FallingSlewLimit=minJerk  SampleTimeMode=inherited
  safe saturation : Saturate  UpperLimit=maxAcceleration  LowerLimit=minAcceleration
  velKi : Gain  Gain=velKi
  velKp : Gain  Gain=velKp
  u : Outport
  errors : Outport  Port=2
  gap : Outport  Port=3
  wires:
  Headway error/1(eh) -> Saturation1/1, Mux/1, Compare To Constant/1
  Bus Selector/2 -> Headway error/2(vf), Sum/1  "<Xdot>"
  Kd/1 -> Scope/3, Sum1/3
  Kp/1 -> Scope/2, Sum1/2
  Gain3/1 -> Saturation/1
  Saturation/1 -> Integrator1/1
  Integrator1/1 -> Sum2/2, Sum/2
  Bus Selector1/2 -> Sum2/1  "<Xdot>"
  Sum2/1 -> Gain3/1
  Saturation1/1 -> Kp/1, Ki/1
  Headway error/2("gap ") -> gap/1
  Integrator2/1 -> velKi/1
  velKi/1 -> Sum3/2
  Switch/1 -> Sum4/1, safe saturation/1, comf saturation/1  "u"
  Sum1/1 -> Switch/1, ACC outputs/1
  Sum3/1 -> ACC outputs/3, Switch/3
  Sum/1 -> Mux/2, Kd/1, velKp/1, Integrator2/1
  Mux/1 -> errors/1
  Sum4/1 -> Anti-windup gain/1
  Sum5/1 -> Integrator/1
  velKp/1 -> Sum3/1
  Ki/1 -> Sum5/2
  Integrator/1 -> Sum1/1, Scope/1
  Anti-windup gain/1 -> Sum5/1
  AND/1 -> Integrator/2, Switch/2, ACC outputs/2
  Compare To Constant/1 -> AND/2
  Compare To Constant1/1 -> AND/1
  lcFlag/1 -> [lcFlag], Headway error/4(lcFlag)
  currentStates/1 -> Bus Selector/1
  Bus Selector/1 -> Headway error/1(xf)  "<X>"
  leaderStates/1 -> Bus Selector1/1
  Bus Selector1/1 -> Compare To Constant1/1, Headway error/3(xl)  "<X>"
  Bus Selector/3 -> [realInput]  "<u>"
  [realInput] -> Sum4/2
  Headway error/3(unsafeFlag) -> [unsafeFlag]
  [unsafeFlag] -> NOT/1
  NOT/1 -> AND1/1
  [lcFlag] -> AND1/2
  AND1/1 -> Switch1/2
  Switch1/1 -> u/1
  safe saturation/1 -> safe jerk/1
  comf saturation/1 -> comf jerk/1
  safe jerk/1 -> Switch1/3  "sat(u)"
  comf jerk/1 -> Switch1/1  "sat(u)"

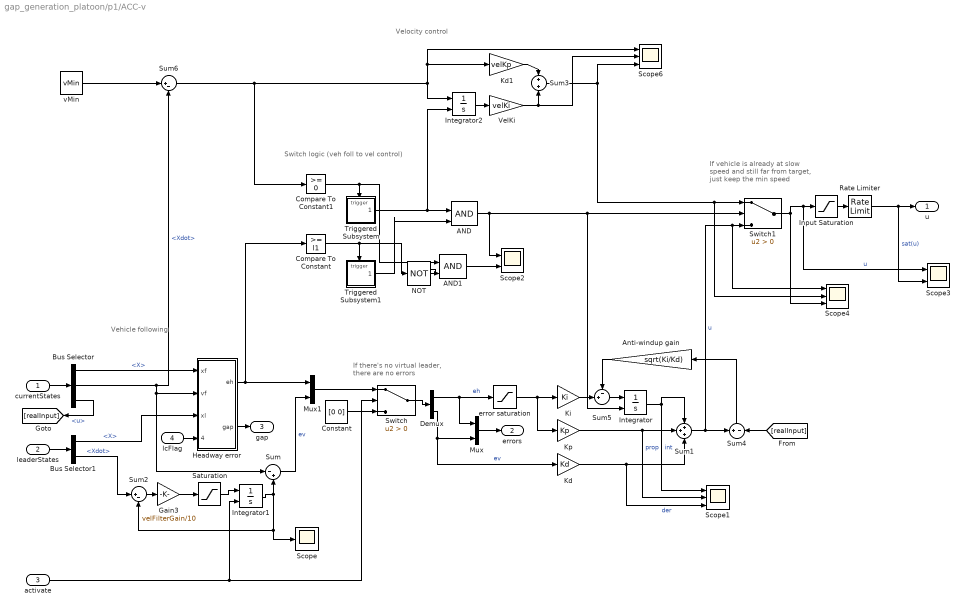
== system gap_generation_platoon/p1/ACC-v ==
  note: Vehicle following
  note: Switch logic (veh foll to vel control)
  note: Velocity control
  note: If vehicle is already at slow
      | speed and still far from target,
      | just keep the min speed
  note: If there's no virtual leader,
      | there are no errors
  currentStates : Inport
  leaderStates : Inport  Port=2
  activate : Inport  Port=3
  lcFlag : Inport  Port=4
  AND : Logic  IconShape=distinctive  AllPortsSameDT=off  OutDataTypeStr=boolean
  AND1 : Logic  IconShape=distinctive  AllPortsSameDT=off  OutDataTypeStr=boolean
  Anti-windup gain : Gain  Gain=sqrt(Ki/Kd)
  Bus Selector : BusSelector  OutputSignals=X,Xdot,u
  Bus Selector1 : BusSelector  OutputSignals=X,Xdot
  Compare To Constant : simulink/Logic and Bit Operations/Compare To Constant  relop=>=  const=l1  OutDataTypeStr=boolean
  Compare To Constant1 : simulink/Logic and Bit Operations/Compare To Constant  relop=>=  const=0  OutDataTypeStr=boolean
  Constant : Constant  Value=[0 0]
  Demux : Demux  Outputs=2
  Gain3 : Gain  Gain=velFilterGain/10
  Headway error : Subsystem
  Input Saturation : Saturate  UpperLimit=maxAcceleration/2  LowerLimit=minAcceleration/4
  Integrator : Integrator  ExternalReset=falling
  Integrator1 : Integrator  ExternalReset=rising  InitialCondition=vx0
  Integrator2 : Integrator  ExternalReset=rising
  Kd : Gain  Gain=Kd
  Kd1 : Gain  Gain=velKp
  Ki : Gain  Gain=Ki
  Kp : Gain  Gain=Kp
  Mux : Mux  Inputs=2
  Mux1 : Mux  Inputs=2
  NOT : Logic  Operator=NOT  IconShape=distinctive  AllPortsSameDT=off  OutDataTypeStr=boolean
  Rate Limiter : RateLimiter  RisingSlewLimit=10  FallingSlewLimit=-10  SampleTimeMode=inherited
  Saturation : Saturate  UpperLimit=maxAcceleration  LowerLimit=minAcceleration
  Scope : Scope
  Scope1 : Scope  NumInputPorts=3
  Scope2 : Scope  NumInputPorts=2
  Scope3 : Scope  NumInputPorts=2
  Scope4 : Scope  NumInputPorts=3
  Scope6 : Scope  NumInputPorts=3
  Sum : Sum  Inputs=|-+
  Sum1 : Sum  Inputs=+++
  Sum2 : Sum  Inputs=|+-
  Sum3 : Sum
  Sum4 : Sum  Inputs=+-
  Sum5 : Sum  Inputs=-+|
  Sum6 : Sum  Inputs=|+-
  Switch : Switch  Criteria=u2 > Threshold
  Switch1 : Switch  Criteria=u2 > Threshold
  Triggered Subsystem : Subsystem  TreatAsAtomicUnit=on
  Triggered Subsystem1 : Subsystem  TreatAsAtomicUnit=on
  VelKi : Gain  Gain=velKi
  error saturation : Saturate  UpperLimit=maxHeadwayError  LowerLimit=minHeadwayError/10
  vMin : Constant  Value=vMin
  u : Outport
  errors : Outport  Port=2
  gap : Outport  Port=3
  wires:
  Headway error/1(eh) -> Mux1/1, Compare To Constant/1
  Kd/1 -> Scope1/3, Sum1/3  "der"
  Kp/1 -> Scope1/2, Sum1/2  "prop"
  Gain3/1 -> Saturation/1
  Saturation/1 -> Integrator1/1
  Integrator1/1 -> Scope/1, Sum2/2, Sum/2
  Bus Selector1/2 -> Sum2/1  "<Xdot>"
  Sum2/1 -> Gain3/1
  Demux/1 -> error saturation/1, Mux/1  "eh"
  Headway error/2("gap ") -> gap/1
  Sum1/1 -> Scope4/1, Switch1/3, Sum4/1  "u"
  Sum/1 -> Mux1/2  "ev"
  Mux/1 -> errors/1
  Input Saturation/1 -> Rate Limiter/1
  Integrator/1 -> Sum1/1, Scope1/1  "int"
  Sum4/1 -> Anti-windup gain/1
  Ki/1 -> Sum5/2
  Anti-windup gain/1 -> Sum5/1
  Demux/2 -> Mux/2, Kd/1  "ev"
  Switch/1 -> Demux/1
  Mux1/1 -> Switch/1
  activate/1 -> Switch/2, Integrator1/2
  Constant/1 -> Switch/3
  Rate Limiter/1 -> Scope3/2, u/1  "sat(u)"
  Compare To Constant1/1 -> AND1/1, Triggered Subsystem/Trigger
  Compare To Constant/1 -> NOT/1, Triggered Subsystem1/Trigger
  Sum6/1 -> Scope6/1, Kd1/1, Integrator2/1, Compare To Constant1/1
  Sum3/1 -> Scope6/3, Scope4/2, Switch1/1
  Integrator2/1 -> VelKi/1
  Kd1/1 -> Sum3/1
  VelKi/1 -> Scope6/2, Sum3/2
  vMin/1 -> Sum6/1
  Switch1/1 -> Scope3/1, Input Saturation/1, Scope4/3  "u"
  error saturation/1 -> Kp/1, Ki/1
  Sum5/1 -> Integrator/1
  Triggered Subsystem/1(Out1) -> AND/1, Integrator2/2
  [realInput] -> Sum4/2
  currentStates/1 -> Bus Selector/1
  Bus Selector/1 -> Headway error/1(xf)  "<X>"
  Bus Selector/2 -> Sum6/2, Headway error/2(vf), Sum/1  "<Xdot>"
  leaderStates/1 -> Bus Selector1/1
  Bus Selector1/1 -> Headway error/3(xl)  "<X>"
  Bus Selector/3 -> [realInput]  "<u>"
  lcFlag/1 -> Headway error/4(lcFlag)
  Triggered Subsystem1/1(Out1) -> AND/2
  AND/1 -> Switch1/2, Integrator/2, Scope2/1
  AND1/1 -> Scope2/2
  NOT/1 -> AND1/2

== system gap_generation_platoon/p1/Detect steady state ==
  errors : Inport
  virtual errors : Inport  Port=2
  ACC-v active : Inport  Port=3
  AND1 : Logic  IconShape=distinctive  AllPortsSameDT=off  OutDataTypeStr=boolean
  AND2 : Logic  IconShape=distinctive  AllPortsSameDT=off  OutDataTypeStr=boolean
  AND5 : Logic  IconShape=distinctive  AllPortsSameDT=off  OutDataTypeStr=boolean
  Abs : Abs
  Abs1 : Abs  ZeroCross=off
  Abs2 : Abs
  Abs3 : Abs  ZeroCross=off
  Compare To Constant{,1..3} (4 alike) : simulink/Logic and Bit Operations/Compare To Constant  relop=<=  const=0.5  OutDataTypeStr=boolean
  Demux : Demux  Outputs=2
  OR : Logic  Operator=OR  IconShape=distinctive  AllPortsSameDT=off  OutDataTypeStr=boolean
  Subsystem : Subsystem
  Transport Delay : TransportDelay
  Transport Delay1 : TransportDelay
  Out1 : Outport
  wires:
  Abs/1 -> Compare To Constant/1
  Transport Delay/1 -> Abs/1
  Abs1/1 -> Compare To Constant1/1
  errors/1 -> Demux/1
  Abs3/1 -> Compare To Constant3/1
  Transport Delay1/1 -> Abs2/1
  Abs2/1 -> Compare To Constant2/1
  Demux/1 -> Abs1/1, Transport Delay/1
  Demux/2 -> Abs3/1, Transport Delay1/1
  Compare To Constant1/1 -> AND1/1
  Compare To Constant/1 -> AND1/2
  Compare To Constant3/1 -> AND2/1
  Compare To Constant2/1 -> AND2/2
  AND1/1 -> AND5/1
  AND2/1 -> AND5/2
  OR/1 -> Out1/1
  AND5/1 -> OR/1
  virtual errors/1 -> Subsystem/1(virtual errors)
  Subsystem/1(Out1) -> OR/2
  ACC-v active/1 -> Subsystem/Enable

== system gap_generation_platoon/p1/Triggered Subsystem ==
  In1 : Inport
  Trigger : TriggerPort  VariantControl=Variant
  Out1 : Outport
  wires:
  In1/1 -> Out1/1
